simulink library "Fixed_Wing"  (R2023b)
settings: Solver=VariableStepAuto  StartTime=0.0  StopTime=10.0  RelTol=1e-3
values from neighbouring files (symbols this model uses):
  X8_lat_da_p_tf = X8_lat_p_tf(1)    [main.m]
  X8_lat_da_r_tf = X8_lat_r_tf(1)    [main.m]
  X8_lon_de_q_tf = X8_lon_q_tf(1)    [main.m]
  X8_lon_th_u_tf = X8_lon_u_tf(2)    [main.m]
  X8_lon_th_w_tf = X8_lon_w_tf(2)    [main.m]
undefined symbols (not defined in the file or in its folder): alpha, beta, env, init, k_phi, k_theta, k_Va, X8
libraries: $bdroot x16, simulink x2
(part 1 of 2)
settings Model: Creator=TigerWuu  LastModifiedBy=NCS

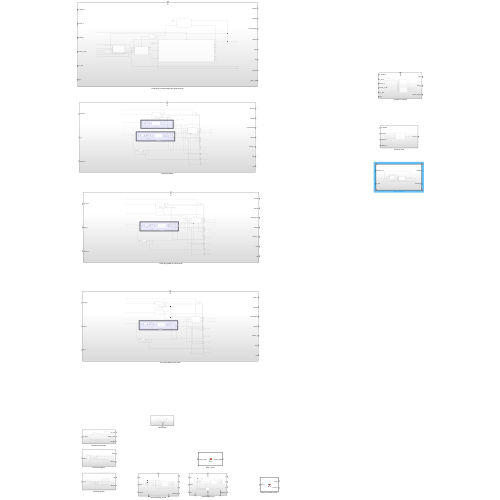
[thumbnail: Simulink's stored preview of the top-level diagram]
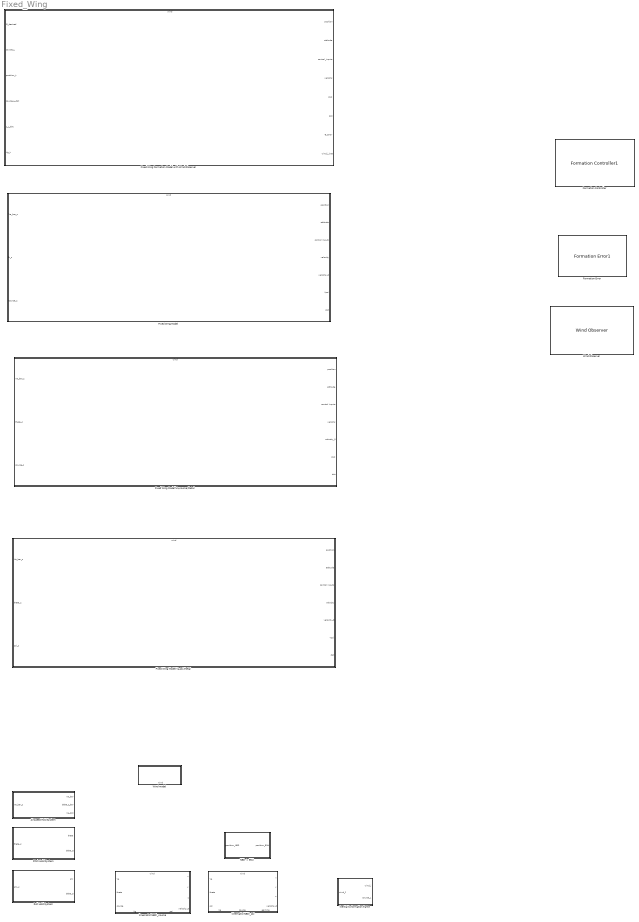
== system Fixed_Wing ==
  Airspeed Hold System : Subsystem
  Fixed Wing Formation Model with Wind Observer : Subsystem
      settings: PortSchema="{\"entries\":[{\"content\":{\"sides\":[{\"content\":{\"connectorIds\":[\"In1\",\"In2\",\"In3\",\"In4\",\"In5\",\"In6\"]},\"type\":\"ConnectorPlacement.EquallySpacedRectSide\",\"uuid\":\"527b8280-b7bb-4bbf-b75e-797629a1d02f\"},{\"content\":{\"connectorIds\":[\"Out1\",\"Out2\",\"Out3\",\"Out4\",\"Out5\",\"Out6\",\"Out7\",\"Out8\"],\"side\":\"RIGHT\"},\"type\":\"ConnectorPlacement.EquallySpacedRectSide\",\"uuid\":\"83651618-4cce-4797-8c5d-5752aadadd0e\"},{\"content\":{\"connectorIds\":[\"In7\"],\"side\":\"TOP\"},\"type\":\"ConnectorPlacement.EquallySpacedRectSide\",\"uuid\":\"91f129b3-c1c6-46ff-9e73-d368da7d167a\"}]},\"type\":\"ConnectorPlacement.EquallySpacedConnector\",\"uuid\":\"d5eae0c8-1f9e-4313-b74c-0f7e22e43491\"}],\"packageUris\":[\"http://schema.mathworks.com/mf0/Connector/R2020b\"],\"version\":\"1.0\"}"
  Fixed Wing Model : Subsystem
      settings: PortSchema="{\"entries\":[{\"content\":{\"sides\":[{\"content\":{\"connectorIds\":[\"In1\",\"In2\",\"In3\"]},\"type\":\"ConnectorPlacement.EquallySpacedRectSide\",\"uuid\":\"491080cc-ba33-4dca-9b37-922a1b131a7c\"},{\"content\":{\"connectorIds\":[\"Out1\",\"Out2\",\"Out3\",\"Out4\",\"Out5\",\"Out6\",\"Out7\"],\"side\":\"RIGHT\"},\"type\":\"ConnectorPlacement.EquallySpacedRectSide\",\"uuid\":\"e4e8ca81-264a-41b3-9d62-a2cb565f7b79\"},{\"content\":{\"connectorIds\":[\"In4\"],\"side\":\"TOP\"},\"type\":\"ConnectorPlacement.EquallySpacedRectSide\",\"uuid\":\"52444ebc-de17-4d3c-95e2-2270054ae63e\"},{\"content\":{\"side\":\"BOTTOM\"},\"type\":\"ConnectorPlacement.EquallySpacedRectSide\",\"uuid\":\"cd38afea-0687-422f-bcb3-a9854084c98f\"}]},\"type\":\"ConnectorPlacement.EquallySpacedConnector\",\"uuid\":\"020d1068-73e8-421c-b651-66bcdf43a07b\"}],\"packageUris\":[\"http://schema.mathworks.com/mf0/Connector/R2020b\"],\"version\":\"1.0\"}"
  Fixed Wing Model(Va,course,theta) : Subsystem
      settings: PortSchema="{\"entries\":[{\"content\":{\"sides\":[{\"content\":{\"connectorIds\":[\"In1\",\"In2\",\"In3\"]},\"type\":\"ConnectorPlacement.EquallySpacedRectSide\",\"uuid\":\"491080cc-ba33-4dca-9b37-922a1b131a7c\"},{\"content\":{\"connectorIds\":[\"Out1\",\"Out2\",\"Out3\",\"Out4\",\"Out5\",\"Out6\",\"Out7\"],\"side\":\"RIGHT\"},\"type\":\"ConnectorPlacement.EquallySpacedRectSide\",\"uuid\":\"e4e8ca81-264a-41b3-9d62-a2cb565f7b79\"},{\"content\":{\"connectorIds\":[\"In4\"],\"side\":\"TOP\"},\"type\":\"ConnectorPlacement.EquallySpacedRectSide\",\"uuid\":\"52444ebc-de17-4d3c-95e2-2270054ae63e\"},{\"content\":{\"side\":\"BOTTOM\"},\"type\":\"ConnectorPlacement.EquallySpacedRectSide\",\"uuid\":\"cd38afea-0687-422f-bcb3-a9854084c98f\"}]},\"type\":\"ConnectorPlacement.EquallySpacedConnector\",\"uuid\":\"020d1068-73e8-421c-b651-66bcdf43a07b\"}],\"packageUris\":[\"http://schema.mathworks.com/mf0/Connector/R2020b\"],\"version\":\"1.0\"}"
  Fixed Wing Model(Va,psi,theta) : Subsystem
      settings: PortSchema="{\"entries\":[{\"content\":{\"sides\":[{\"content\":{\"connectorIds\":[\"In1\",\"In2\",\"In3\"]},\"type\":\"ConnectorPlacement.EquallySpacedRectSide\",\"uuid\":\"491080cc-ba33-4dca-9b37-922a1b131a7c\"},{\"content\":{\"connectorIds\":[\"Out1\",\"Out2\",\"Out3\",\"Out4\",\"Out5\",\"Out6\",\"Out7\"],\"side\":\"RIGHT\"},\"type\":\"ConnectorPlacement.EquallySpacedRectSide\",\"uuid\":\"e4e8ca81-264a-41b3-9d62-a2cb565f7b79\"},{\"content\":{\"connectorIds\":[\"In4\"],\"side\":\"TOP\"},\"type\":\"ConnectorPlacement.EquallySpacedRectSide\",\"uuid\":\"52444ebc-de17-4d3c-95e2-2270054ae63e\"},{\"content\":{\"side\":\"BOTTOM\"},\"type\":\"ConnectorPlacement.EquallySpacedRectSide\",\"uuid\":\"cd38afea-0687-422f-bcb3-a9854084c98f\"}]},\"type\":\"ConnectorPlacement.EquallySpacedConnector\",\"uuid\":\"020d1068-73e8-421c-b651-66bcdf43a07b\"}],\"packageUris\":[\"http://schema.mathworks.com/mf0/Connector/R2020b\"],\"version\":\"1.0\"}"
  Formation Controller : $bdroot/Fixed Wing Formation Model with Wind Observer/Formation Controller1  SystemSampleTime=-1  VariantActivationTime=update diagram  AllowFlexibleInterface=on  Latency=0  AutoFrameSizeCalculation=off
      settings: PortSchema="{\"entries\":[{\"content\":{\"sides\":[{\"content\":{\"connectorIds\":[\"In1\",\"In2\",\"In3\",\"In4\",\"In5\",\"In6\"]},\"type\":\"ConnectorPlacement.EquallySpacedRectSide\",\"uuid\":\"9c389f85-23f7-4ad0-9870-58a1e0934639\"},{\"content\":{\"connectorIds\":[\"Out1\",\"Out2\",\"Out3\"],\"side\":\"RIGHT\"},\"type\":\"ConnectorPlacement.EquallySpacedRectSide\",\"uuid\":\"ce3247c4-1bae-44d3-b9da-13662f8788fa\"},{\"content\":{\"connectorIds\":[\"In7\"],\"side\":\"TOP\"},\"type\":\"ConnectorPlacement.EquallySpacedRectSide\",\"uuid\":\"1a627aed-9846-48b6-b280-b2fda66f57fb\"}]},\"type\":\"ConnectorPlacement.EquallySpacedConnector\",\"uuid\":\"4ccca4c3-7c97-47a5-8a1e-b96349422d36\"}],\"packageUris\":[\"http://schema.mathworks.com/mf0/Connector/R2020b\"],\"version\":\"1.0\"}"
  Formation Error : $bdroot/Fixed Wing Formation Model with Wind Observer/Formation Error1  SystemSampleTime=-1  VariantActivationTime=update diagram  AllowFlexibleInterface=on  Latency=0  AutoFrameSizeCalculation=off
  Inertial to formation frame : MATLAB Function  TreatAsAtomicUnit=on
  "NED -> ENU" : MATLAB Function  TreatAsAtomicUnit=on
  "Pitch Hold System " : Subsystem
      settings: ModelCloseFcn=function
  Roll Hold System : Subsystem
      settings: ModelCloseFcn=function
  Wind Observer : $bdroot/Fixed Wing Formation Model with Wind Observer/Wind Observer  SystemSampleTime=-1  VariantActivationTime=update diagram  AllowFlexibleInterface=on  Latency=0  AutoFrameSizeCalculation=off
  Wind model : Subsystem
      settings: PortSchema="{\"entries\":[{\"content\":{\"sides\":[{\"content\":{},\"type\":\"ConnectorPlacement.EquallySpacedRectSide\",\"uuid\":\"19ef0eb7-c626-45ec-b76b-8668fc024824\"},{\"content\":{\"side\":\"RIGHT\"},\"type\":\"ConnectorPlacement.EquallySpacedRectSide\",\"uuid\":\"89e72569-ab94-4162-a6e2-b425ef08f724\"},{\"content\":{\"side\":\"TOP\"},\"type\":\"ConnectorPlacement.EquallySpacedRectSide\",\"uuid\":\"6d9409e9-6822-4cd9-902f-e5665cb68433\"},{\"content\":{\"connectorIds\":[\"Out1\"],\"side\":\"BOTTOM\"},\"type\":\"ConnectorPlacement.EquallySpacedRectSide\",\"uuid\":\"39a83352-0924-44fa-be5d-94a7c28bbbf3\"}]},\"type\":\"ConnectorPlacement.EquallySpacedConnector\",\"uuid\":\"6cf6ae00-ef23-42a2-99b2-ca60e191fb03\"}],\"packageUris\":[\"http://schema.mathworks.com/mf0/Connector/R2020b\"],\"version\":\"1.0\"}"
  kinematic(NED)_course : Subsystem
      settings: PortSchema="{\"entries\":[{\"content\":{\"sides\":[{\"content\":{\"connectorIds\":[\"In1\",\"In2\",\"In3\"]},\"type\":\"ConnectorPlacement.EquallySpacedRectSide\",\"uuid\":\"96d967d8-b822-4ab1-b08a-27adc20d5833\"},{\"content\":{\"connectorIds\":[\"Out1\",\"Out2\",\"Out3\",\"Out4\"],\"side\":\"RIGHT\"},\"type\":\"ConnectorPlacement.EquallySpacedRectSide\",\"uuid\":\"505a36c9-cae2-422c-97bf-34d37872a31d\"},{\"content\":{\"connectorIds\":[\"In4\"],\"side\":\"TOP\"},\"type\":\"ConnectorPlacement.EquallySpacedRectSide\",\"uuid\":\"7bc53155-5df6-4b6a-9756-725497693b0a\"},{\"content\":{\"connectorIds\":[\"Out5\",\"Out6\"],\"side\":\"BOTTOM\"},\"type\":\"ConnectorPlacement.EquallySpacedRectSide\",\"uuid\":\"7777b465-a27e-4b61-9b89-f3b8fa4654d1\"}]},\"type\":\"ConnectorPlacement.EquallySpacedConnector\",\"uuid\":\"2150a812-5a4a-4a29-9c93-d226d95b2326\"}],\"packageUris\":[\"http://schema.mathworks.com/mf0/Connector/R2020b\"],\"version\":\"1.0\"}"
  kinematic(NED)_psi : Subsystem
      settings: PortSchema="{\"entries\":[{\"content\":{\"sides\":[{\"content\":{\"connectorIds\":[\"In1\",\"In2\",\"In3\"]},\"type\":\"ConnectorPlacement.EquallySpacedRectSide\",\"uuid\":\"96d967d8-b822-4ab1-b08a-27adc20d5833\"},{\"content\":{\"connectorIds\":[\"Out1\",\"Out2\",\"Out3\",\"Out4\"],\"side\":\"RIGHT\"},\"type\":\"ConnectorPlacement.EquallySpacedRectSide\",\"uuid\":\"505a36c9-cae2-422c-97bf-34d37872a31d\"},{\"content\":{\"connectorIds\":[\"In4\"],\"side\":\"TOP\"},\"type\":\"ConnectorPlacement.EquallySpacedRectSide\",\"uuid\":\"7bc53155-5df6-4b6a-9756-725497693b0a\"},{\"content\":{\"connectorIds\":[\"Out5\",\"Out6\",\"Out7\"],\"side\":\"BOTTOM\"},\"type\":\"ConnectorPlacement.EquallySpacedRectSide\",\"uuid\":\"7777b465-a27e-4b61-9b89-f3b8fa4654d1\"}]},\"type\":\"ConnectorPlacement.EquallySpacedConnector\",\"uuid\":\"2150a812-5a4a-4a29-9c93-d226d95b2326\"}],\"packageUris\":[\"http://schema.mathworks.com/mf0/Connector/R2020b\"],\"version\":\"1.0\"}"

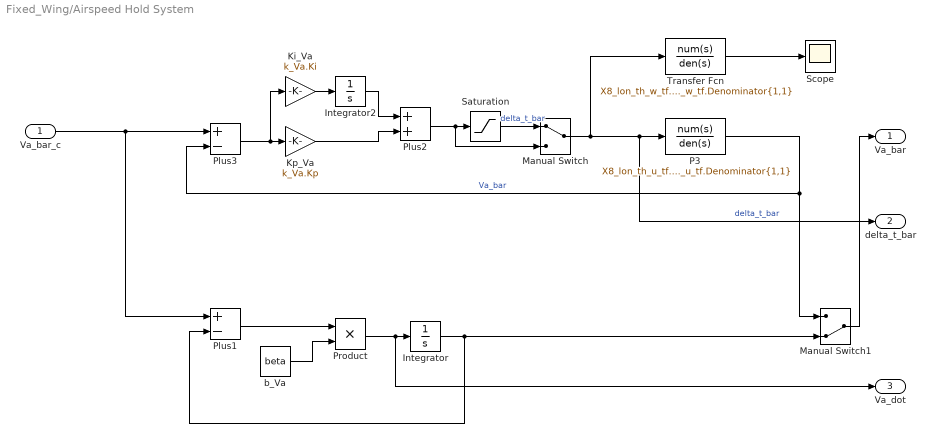
== system Fixed_Wing/Airspeed Hold System ==
  Va_bar_c : Inport
  Integrator : Integrator
  Integrator2 : Integrator
  Ki_Va : Gain  Gain=k_Va.Ki
  Kp_Va : Gain  Gain=k_Va.Kp
  Manual Switch : ManualSwitch
  Manual Switch1 : ManualSwitch  CurrentSetting=0
  P3 : TransferFcn  Numerator=X8_lon_th_u_tf.Numerator{1,1}  Denominator=X8_lon_th_u_tf.Denominator{1,1}
  Plus1 : Sum  Inputs=+-
  Plus2 : Sum
  Plus3 : Sum  Inputs=+-
  Product : Product
  Saturation : Saturate  UpperLimit=X8.delta.t_max-X8.delta.t_star  LowerLimit=X8.delta.t_min -X8.delta.t_star  LinearizeAsGain=off
  Scope : Scope
  Transfer Fcn : TransferFcn  Numerator=X8_lon_th_w_tf.Numerator{1,1}  Denominator=X8_lon_th_w_tf.Denominator{1,1}
  b_Va : Constant  Value=beta
  Va_bar : Outport
  delta_t_bar : Outport  Port=2
  Va_dot : Outport  Port=3
  wires:
  Ki_Va/1 -> Integrator2/1
  Plus3/1 -> Ki_Va/1, Kp_Va/1
  Kp_Va/1 -> Plus2/2
  Plus2/1 -> Manual Switch/2, Saturation/1
  Integrator2/1 -> Plus2/1
  P3/1 -> Manual Switch1/1, Plus3/2  "Va_bar"
  Manual Switch/1 -> Transfer Fcn/1, P3/1, delta_t_bar/1  "delta_t_bar"
  Transfer Fcn/1 -> Scope/1
  Saturation/1 -> Manual Switch/1  "delta_t_bar"
  Plus1/1 -> Product/1
  b_Va/1 -> Product/2
  Product/1 -> Va_dot/1, Integrator/1
  Integrator/1 -> Manual Switch1/2, Plus1/2
  Va_bar_c/1 -> Plus1/1, Plus3/1
  Manual Switch1/1 -> Va_bar/1

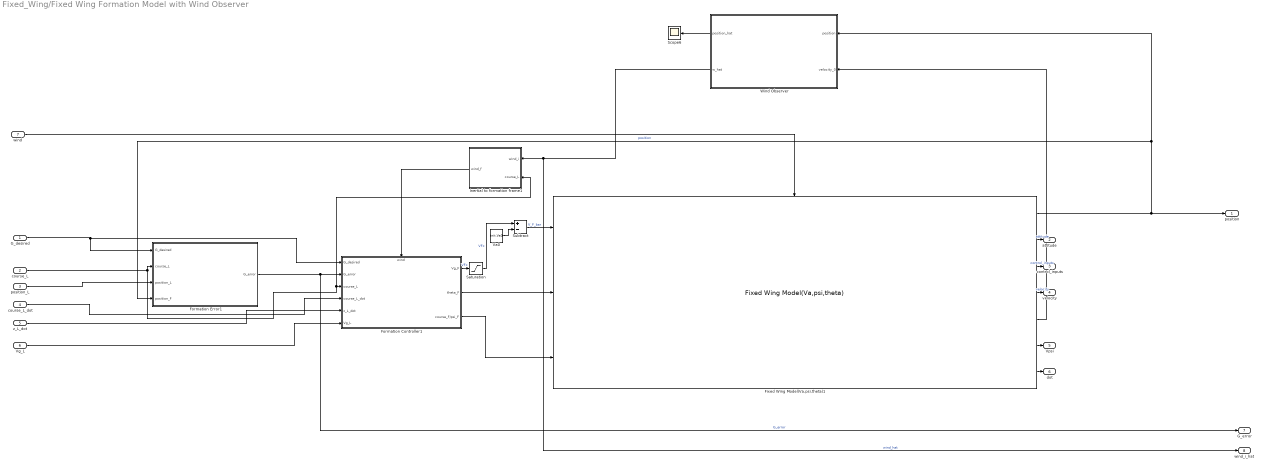
== system Fixed_Wing/Fixed Wing Formation Model with Wind Observer ==
  G_desired : Inport
  course_L : Inport  Port=2
  position_L : Inport  Port=3
  course_L_dot : Inport  Port=4
  z_L_dot : Inport  Port=5
  Vg_L : Inport  Port=6
  wind : Inport  Port=7
  Fixed Wing Model(Va,psi,theta)1 : $bdroot/Fixed Wing Model(Va,psi,theta)  SystemSampleTime=-1  VariantActivationTime=update diagram  AllowFlexibleInterface=on  Latency=0  AutoFrameSizeCalculation=off
      link override Ki_course: Gain=0
      settings: PortSchema="{\"entries\":[{\"content\":{\"sides\":[{\"content\":{\"connectorIds\":[\"In1\",\"In2\",\"In3\"]},\"type\":\"ConnectorPlacement.EquallySpacedRectSide\",\"uuid\":\"491080cc-ba33-4dca-9b37-922a1b131a7c\"},{\"content\":{\"connectorIds\":[\"Out1\",\"Out2\",\"Out3\",\"Out4\",\"Out5\",\"Out6\",\"Out7\"],\"side\":\"RIGHT\"},\"type\":\"ConnectorPlacement.EquallySpacedRectSide\",\"uuid\":\"e4e8ca81-264a-41b3-9d62-a2cb565f7b79\"},{\"content\":{\"connectorIds\":[\"In4\"],\"side\":\"TOP\"},\"type\":\"ConnectorPlacement.EquallySpacedRectSide\",\"uuid\":\"52444ebc-de17-4d3c-95e2-2270054ae63e\"},{\"content\":{\"side\":\"BOTTOM\"},\"type\":\"ConnectorPlacement.EquallySpacedRectSide\",\"uuid\":\"cd38afea-0687-422f-bcb3-a9854084c98f\"}]},\"type\":\"ConnectorPlacement.EquallySpacedConnector\",\"uuid\":\"020d1068-73e8-421c-b651-66bcdf43a07b\"}],\"packageUris\":[\"http://schema.mathworks.com/mf0/Connector/R2020b\"],\"version\":\"1.0\"}"
  Formation Controller1 : Subsystem
      settings: PortSchema="{\"entries\":[{\"content\":{\"sides\":[{\"content\":{\"connectorIds\":[\"In1\",\"In2\",\"In3\",\"In4\",\"In5\",\"In6\"]},\"type\":\"ConnectorPlacement.EquallySpacedRectSide\",\"uuid\":\"9c389f85-23f7-4ad0-9870-58a1e0934639\"},{\"content\":{\"connectorIds\":[\"Out1\",\"Out2\",\"Out3\"],\"side\":\"RIGHT\"},\"type\":\"ConnectorPlacement.EquallySpacedRectSide\",\"uuid\":\"ce3247c4-1bae-44d3-b9da-13662f8788fa\"},{\"content\":{\"connectorIds\":[\"In7\"],\"side\":\"TOP\"},\"type\":\"ConnectorPlacement.EquallySpacedRectSide\",\"uuid\":\"1a627aed-9846-48b6-b280-b2fda66f57fb\"}]},\"type\":\"ConnectorPlacement.EquallySpacedConnector\",\"uuid\":\"4ccca4c3-7c97-47a5-8a1e-b96349422d36\"}],\"packageUris\":[\"http://schema.mathworks.com/mf0/Connector/R2020b\"],\"version\":\"1.0\"}"
  Formation Error1 : Subsystem
  Inertial to formation frame1 : MATLAB Function  TreatAsAtomicUnit=on
  Saturation : Saturate  UpperLimit=28  LowerLimit=12
  Scope6 : Scope
  Subtract : Sum  Inputs=+-
  Va0 : Constant  Value=init.Va0
  Wind Observer : Subsystem
  position : Outport
  attitude : Outport  Port=2
  control_inputs : Outport  Port=3
  velocity : Outport  Port=4
  Vpsi : Outport  Port=5
  dot : Outport  Port=6
  G_error : Outport  Port=7
  wind_i_hat : Outport  Port=8
  wires:
  Wind Observer/1(position_hat) -> Scope6/1
  Va0/1 -> Subtract/2
  Fixed Wing Model(Va,psi,theta)1/2 -> attitude/1  "attitude"
  Fixed Wing Model(Va,psi,theta)1/1 -> position/1, Formation Error1/4(position_F), Wind Observer/1(position)  "position"
  wind/1 -> Fixed Wing Model(Va,psi,theta)1/4
  position_L/1 -> Formation Error1/3(position_L)
  Vg_L/1 -> Formation Controller1/6(Vg_L)
  Fixed Wing Model(Va,psi,theta)1/7 -> dot/1
  Formation Controller1/2(theta_F) -> Fixed Wing Model(Va,psi,theta)1/2
  Formation Error1/1(G_error) -> G_error/1, Formation Controller1/2(G_error)  "G_error"
  Formation Controller1/1(Vg_F) -> Saturation/1  "VFc"
  Subtract/1 -> Fixed Wing Model(Va,psi,theta)1/1  "V_F_bar"
  Formation Controller1/3(course_F/psi_F) -> Fixed Wing Model(Va,psi,theta)1/3
  Fixed Wing Model(Va,psi,theta)1/3 -> control_inputs/1  "control_inputs"
  Wind Observer/2(w_hat) -> wind_i_hat/1, Inertial to formation frame1/1(wind_i)  "wind_hat"
  course_L/1 -> Inertial to formation frame1/2(course_L), Formation Controller1/3(course_L), Formation Error1/2(course_L)
  Fixed Wing Model(Va,psi,theta)1/4 -> velocity/1  "velocity"
  Inertial to formation frame1/1(wind_f) -> Formation Controller1/7(wind)
  Saturation/1 -> Subtract/1  "VFc"
  Fixed Wing Model(Va,psi,theta)1/5 -> Wind Observer/2(velocity_0)
  z_L_dot/1 -> Formation Controller1/5(z_L_dot)
  course_L_dot/1 -> Formation Controller1/4(course_L_dot)
  G_desired/1 -> Formation Error1/1(G_desired), Formation Controller1/1(G_desired)
  Fixed Wing Model(Va,psi,theta)1/6 -> Vpsi/1

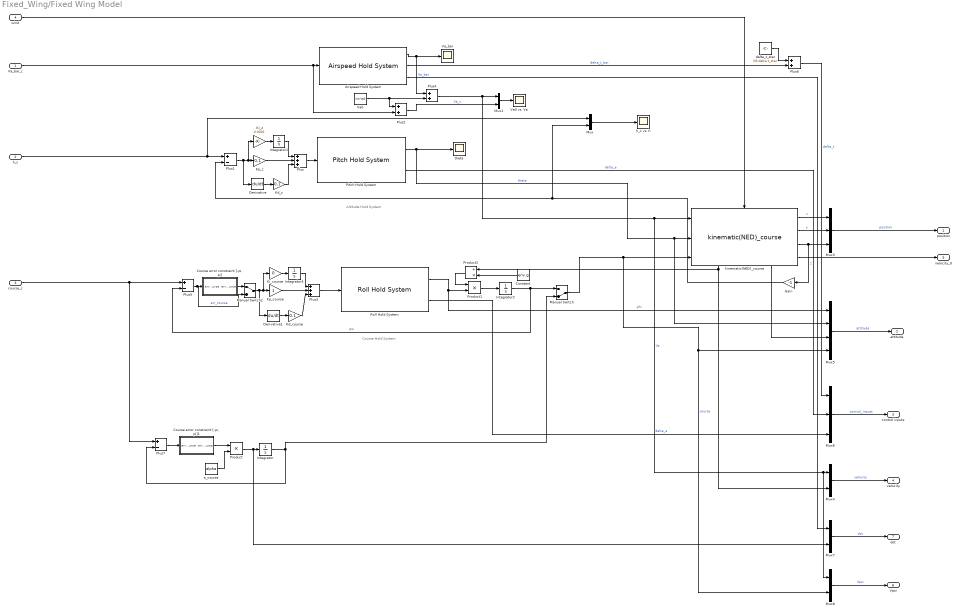
== system Fixed_Wing/Fixed Wing Model ==
  note: Course Hold System
  note: Altitude Hold System
  Va_bar_c : Inport
  h_c : Inport  Port=2
  course_c : Inport  Port=3
  wind : Inport  Port=4
  Airspeed Hold System : $bdroot/Airspeed Hold System  SystemSampleTime=-1  VariantActivationTime=update diagram  AllowFlexibleInterface=on  Latency=0  AutoFrameSizeCalculation=off
      link override b_Va: Value=beta
  Constant : Constant  Value=env.g
  "Course error constraint [-pi, pi]" : MATLAB Function  TreatAsAtomicUnit=on
  "Course error constraint [-pi, pi]1" : MATLAB Function  TreatAsAtomicUnit=on
  Derivative : Derivative
  Derivative1 : Derivative
  Gain : Gain  Gain=-1
  Integrator : Integrator
  Integrator1 : Integrator
  Integrator2 : Integrator  InitialCondition=init.course0
  Integrator3 : Integrator
  Kd_course : Gain  Gain=0.1
  Kd_z : Gain  Gain=0.1
  Ki_course : Gain  Gain=0
  Ki_z : Gain  Gain=0.0001
  Kp_course : Gain
  Kp_z : Gain  Gain=0.1
  Manual Switch : ManualSwitch  CurrentSetting=0
  Manual Switch2 : ManualSwitch
  Mux{,1,4,7..8} (5 alike) : Mux  Inputs=2
  Mux3 : Mux  Inputs=3
  Mux5 : Mux
  Mux6 : Mux  Inputs=3
  "Pitch Hold System " : $bdroot/Pitch Hold System   SystemSampleTime=-1  VariantActivationTime=update diagram  AllowFlexibleInterface=on  Latency=0  AutoFrameSizeCalculation=off
  Plus : Sum  Inputs=+++
  Plus1 : Sum  Inputs=+-
  Plus2 : Sum
  Plus3 : Sum  Inputs=+++
  Plus4 : Sum
  Plus5 : Sum  Inputs=+-
  Plus6 : Sum
  Plus7 : Sum  Inputs=+-
  Product : Product
  Product1 : Product
  Product2 : Product  Inputs=/*
  Roll Hold System : $bdroot/Roll Hold System  SystemSampleTime=-1  VariantActivationTime=update diagram  AllowFlexibleInterface=on  Latency=0  AutoFrameSizeCalculation=off
  Va0 : Constant  Value=init.Va0
  Va0 vs. Va : Scope
  Va_bar : Scope
  a_course : Constant  Value=alpha
  delta_t_star : Constant  Value=X8.delta.t_star
  h_c vs. h : Scope
  kinematic(NED)_course : $bdroot/kinematic(NED)_course  SystemSampleTime=-1  VariantActivationTime=update diagram  AllowFlexibleInterface=on  Latency=0  AutoFrameSizeCalculation=off
      settings: PortSchema="{\"entries\":[{\"content\":{\"sides\":[{\"content\":{\"connectorIds\":[\"In1\",\"In2\",\"In3\"]},\"type\":\"ConnectorPlacement.EquallySpacedRectSide\",\"uuid\":\"96d967d8-b822-4ab1-b08a-27adc20d5833\"},{\"content\":{\"connectorIds\":[\"Out1\",\"Out2\",\"Out3\",\"Out4\"],\"side\":\"RIGHT\"},\"type\":\"ConnectorPlacement.EquallySpacedRectSide\",\"uuid\":\"505a36c9-cae2-422c-97bf-34d37872a31d\"},{\"content\":{\"connectorIds\":[\"In4\"],\"side\":\"TOP\"},\"type\":\"ConnectorPlacement.EquallySpacedRectSide\",\"uuid\":\"7bc53155-5df6-4b6a-9756-725497693b0a\"},{\"content\":{\"connectorIds\":[\"Out5\",\"Out6\"],\"side\":\"BOTTOM\"},\"type\":\"ConnectorPlacement.EquallySpacedRectSide\",\"uuid\":\"7777b465-a27e-4b61-9b89-f3b8fa4654d1\"}]},\"type\":\"ConnectorPlacement.EquallySpacedConnector\",\"uuid\":\"2150a812-5a4a-4a29-9c93-d226d95b2326\"}],\"packageUris\":[\"http://schema.mathworks.com/mf0/Connector/R2020b\"],\"version\":\"1.0\"}"
  theta : Scope
  position : Outport
  attitude : Outport  Port=2
  control inputs : Outport  Port=3
  velocity : Outport  Port=4
  velocity_0 : Outport  Port=5
  Vpsi : Outport  Port=6
  dot : Outport  Port=7
  wires:
  Integrator3/1 -> Plus3/1
  Integrator1/1 -> Plus/1
  kinematic(NED)_course/3 -> Gain/1, Mux3/3  "z"
  kinematic(NED)_course/1 -> Mux3/1  "x"
  Derivative1/1 -> Kd_course/1
  Constant/1 -> Product2/2
  Va0/1 -> Plus2/1, Plus4/2
  "Pitch Hold System "/1 -> kinematic(NED)_course/2, Mux5/2, theta/1  "theta"
  Kd_z/1 -> Plus/3
  kinematic(NED)_course/2 -> Mux3/2  "y"
  h_c/1 -> Mux/1, Plus1/1
  Plus1/1 -> Derivative/1, Ki_z/1, Kp_z/1
  Va_bar_c/1 -> Plus2/2, Airspeed Hold System/1
  Gain/1 -> Mux/2, Plus1/2
  Roll Hold System/2 -> Mux6/3  "delta_a"
  Kp_z/1 -> Plus/2
  Plus/1 -> "Pitch Hold System "/1
  Airspeed Hold System/2 -> Plus6/2  "delta_t_bar"
  Derivative/1 -> Kd_z/1
  "Pitch Hold System "/2 -> Mux6/2  "delta_e"
  Plus6/1 -> Mux6/1  "delta_t"
  Airspeed Hold System/1 -> Plus4/1, Va_bar/1  "Va_bar"
  delta_t_star/1 -> Plus6/1
  Mux3/1 -> position/1  "position"
  Ki_z/1 -> Integrator1/1
  Integrator2/1 -> Manual Switch/1, Plus5/2  "psi"
  Ki_course/1 -> Integrator3/1
  Product1/1 -> Integrator2/1
  Kp_course/1 -> Plus3/2
  Product2/1 -> Product1/1
  Plus5/1 -> Manual Switch2/2, "Course error constraint [-pi, pi]"/1("err_course ")  "err_course"
  Plus3/1 -> Roll Hold System/1
  Mux/1 -> h_c vs. h/1
  Plus4/1 -> Mux1/1, kinematic(NED)_course/1, Mux8/1, Mux4/1  "Va"
  Mux1/1 -> Va0 vs. Va/1
  kinematic(NED)_course/5 -> Mux4/2, Product2/1
  Mux6/1 -> control inputs/1  "control_inputs"
  Plus2/1 -> Mux1/2  "Va_c"
  Mux5/1 -> attitude/1  "attitude"
  Kd_course/1 -> Plus3/3
  Roll Hold System/1 -> Mux5/1, Product1/2  "phi"
  wind/1 -> kinematic(NED)_course/4
  Manual Switch2/1 -> Derivative1/1, Ki_course/1, Kp_course/1
  Mux4/1 -> velocity/1  "velocity"
  "Course error constraint [-pi, pi]"/1(err_course) -> Manual Switch2/1
  a_course/1 -> Product/2
  Product/1 -> Mux7/2, Integrator/1
  Integrator/1 -> Manual Switch/2, Plus7/2
  Plus7/1 -> "Course error constraint [-pi, pi]1"/1("err_course ")
  course_c/1 -> Plus5/1, Plus7/1
  "Course error constraint [-pi, pi]1"/1(err_course) -> Product/1
  Mux7/1 -> dot/1  "dot"
  Airspeed Hold System/3 -> Mux7/1
  Mux8/1 -> Vpsi/1  "Vpsi"
  Manual Switch/1 -> kinematic(NED)_course/3, Mux8/2, Mux5/4  "course"
  kinematic(NED)_course/4 -> velocity_0/1
  kinematic(NED)_course/6 -> Mux5/3

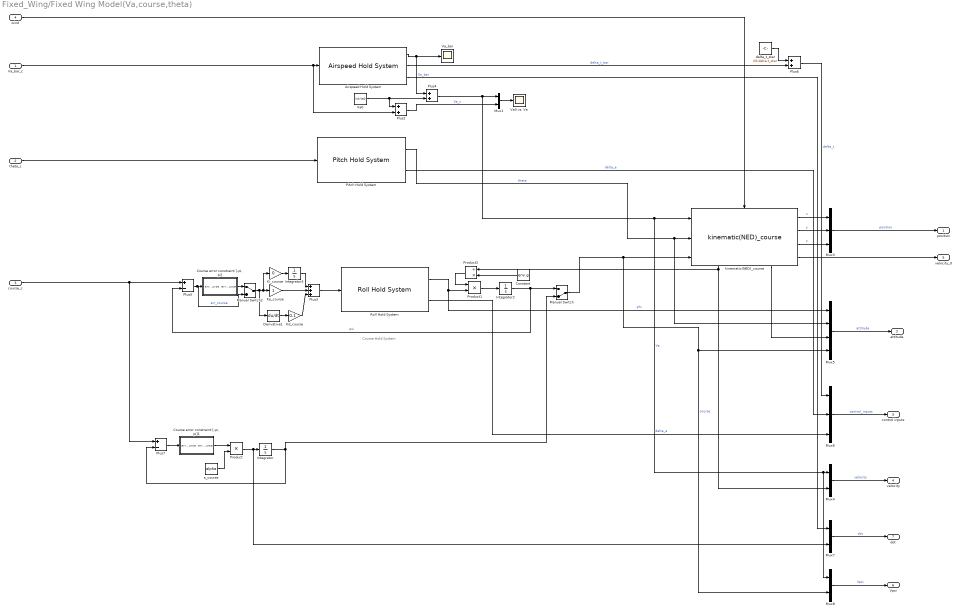
== system Fixed_Wing/Fixed Wing Model(Va,course,theta) ==
  note: Course Hold System
  Va_bar_c : Inport
  theta_c : Inport  Port=2
  course_c : Inport  Port=3
  wind : Inport  Port=4
  Airspeed Hold System : $bdroot/Airspeed Hold System  SystemSampleTime=-1  VariantActivationTime=update diagram  AllowFlexibleInterface=on  Latency=0  AutoFrameSizeCalculation=off
  Constant : Constant  Value=env.g
  "Course error constraint [-pi, pi]" : MATLAB Function  TreatAsAtomicUnit=on
  "Course error constraint [-pi, pi]1" : MATLAB Function  TreatAsAtomicUnit=on
  Derivative1 : Derivative
  Integrator : Integrator
  Integrator2 : Integrator  InitialCondition=init.course0
  Integrator3 : Integrator
  Kd_course : Gain  Gain=0.1
  Ki_course : Gain  Gain=0
  Kp_course : Gain
  Manual Switch : ManualSwitch  CurrentSetting=0
  Manual Switch2 : ManualSwitch
  Mux{1,4,7..8} (4 alike) : Mux  Inputs=2
  Mux3 : Mux  Inputs=3
  Mux5 : Mux
  Mux6 : Mux  Inputs=3
  "Pitch Hold System " : $bdroot/Pitch Hold System   SystemSampleTime=-1  VariantActivationTime=update diagram  AllowFlexibleInterface=on  Latency=0  AutoFrameSizeCalculation=off
  Plus2 : Sum
  Plus3 : Sum  Inputs=+++
  Plus4 : Sum
  Plus5 : Sum  Inputs=+-
  Plus6 : Sum
  Plus7 : Sum  Inputs=+-
  Product : Product
  Product1 : Product
  Product2 : Product  Inputs=/*
  Roll Hold System : $bdroot/Roll Hold System  SystemSampleTime=-1  VariantActivationTime=update diagram  AllowFlexibleInterface=on  Latency=0  AutoFrameSizeCalculation=off
  Va0 : Constant  Value=init.Va0
  Va0 vs. Va : Scope
  Va_bar : Scope
  a_course : Constant  Value=alpha
  delta_t_star : Constant  Value=X8.delta.t_star
  kinematic(NED)_course : $bdroot/kinematic(NED)_course  SystemSampleTime=-1  VariantActivationTime=update diagram  AllowFlexibleInterface=on  Latency=0  AutoFrameSizeCalculation=off
      settings: PortSchema="{\"entries\":[{\"content\":{\"sides\":[{\"content\":{\"connectorIds\":[\"In1\",\"In2\",\"In3\"]},\"type\":\"ConnectorPlacement.EquallySpacedRectSide\",\"uuid\":\"96d967d8-b822-4ab1-b08a-27adc20d5833\"},{\"content\":{\"connectorIds\":[\"Out1\",\"Out2\",\"Out3\",\"Out4\"],\"side\":\"RIGHT\"},\"type\":\"ConnectorPlacement.EquallySpacedRectSide\",\"uuid\":\"505a36c9-cae2-422c-97bf-34d37872a31d\"},{\"content\":{\"connectorIds\":[\"In4\"],\"side\":\"TOP\"},\"type\":\"ConnectorPlacement.EquallySpacedRectSide\",\"uuid\":\"7bc53155-5df6-4b6a-9756-725497693b0a\"},{\"content\":{\"connectorIds\":[\"Out5\",\"Out6\"],\"side\":\"BOTTOM\"},\"type\":\"ConnectorPlacement.EquallySpacedRectSide\",\"uuid\":\"7777b465-a27e-4b61-9b89-f3b8fa4654d1\"}]},\"type\":\"ConnectorPlacement.EquallySpacedConnector\",\"uuid\":\"2150a812-5a4a-4a29-9c93-d226d95b2326\"}],\"packageUris\":[\"http://schema.mathworks.com/mf0/Connector/R2020b\"],\"version\":\"1.0\"}"
  position : Outport
  attitude : Outport  Port=2
  control inputs : Outport  Port=3
  velocity : Outport  Port=4
  velocity_0 : Outport  Port=5
  Vpsi : Outport  Port=6
  dot : Outport  Port=7
  wires:
  Integrator3/1 -> Plus3/1
  kinematic(NED)_course/3 -> Mux3/3  "z"
  kinematic(NED)_course/1 -> Mux3/1  "x"
  Derivative1/1 -> Kd_course/1
  Constant/1 -> Product2/2
  Va0/1 -> Plus2/1, Plus4/2
  "Pitch Hold System "/1 -> kinematic(NED)_course/2, Mux5/2  "theta"
  kinematic(NED)_course/2 -> Mux3/2  "y"
  Va_bar_c/1 -> Plus2/2, Airspeed Hold System/1
  Roll Hold System/2 -> Mux6/3  "delta_a"
  theta_c/1 -> "Pitch Hold System "/1
  Airspeed Hold System/2 -> Plus6/2  "delta_t_bar"
  "Pitch Hold System "/2 -> Mux6/2  "delta_e"
  Plus6/1 -> Mux6/1  "delta_t"
  Airspeed Hold System/1 -> Plus4/1, Va_bar/1  "Va_bar"
  delta_t_star/1 -> Plus6/1
  Mux3/1 -> position/1  "position"
  Integrator2/1 -> Manual Switch/1, Plus5/2  "psi"
  Ki_course/1 -> Integrator3/1
  Product1/1 -> Integrator2/1
  Kp_course/1 -> Plus3/2
  Product2/1 -> Product1/1
  Plus5/1 -> Manual Switch2/2, "Course error constraint [-pi, pi]"/1("err_course ")  "err_course"
  Plus3/1 -> Roll Hold System/1
  Plus4/1 -> Mux1/1, kinematic(NED)_course/1, Mux8/1, Mux4/1  "Va"
  Mux1/1 -> Va0 vs. Va/1
  kinematic(NED)_course/5 -> Mux4/2, Product2/1
  Mux6/1 -> control inputs/1  "control_inputs"
  Plus2/1 -> Mux1/2  "Va_c"
  Mux5/1 -> attitude/1  "attitude"
  Kd_course/1 -> Plus3/3
  Roll Hold System/1 -> Mux5/1, Product1/2  "phi"
  wind/1 -> kinematic(NED)_course/4
  Manual Switch2/1 -> Derivative1/1, Ki_course/1, Kp_course/1
  Mux4/1 -> velocity/1  "velocity"
  "Course error constraint [-pi, pi]"/1(err_course) -> Manual Switch2/1
  a_course/1 -> Product/2
  Product/1 -> Mux7/2, Integrator/1
  Integrator/1 -> Manual Switch/2, Plus7/2
  Plus7/1 -> "Course error constraint [-pi, pi]1"/1("err_course ")
  course_c/1 -> Plus5/1, Plus7/1
  "Course error constraint [-pi, pi]1"/1(err_course) -> Product/1
  Mux7/1 -> dot/1  "dot"
  Airspeed Hold System/3 -> Mux7/1
  Mux8/1 -> Vpsi/1  "Vpsi"
  Manual Switch/1 -> kinematic(NED)_course/3, Mux8/2, Mux5/4  "course"
  kinematic(NED)_course/4 -> velocity_0/1
  kinematic(NED)_course/6 -> Mux5/3

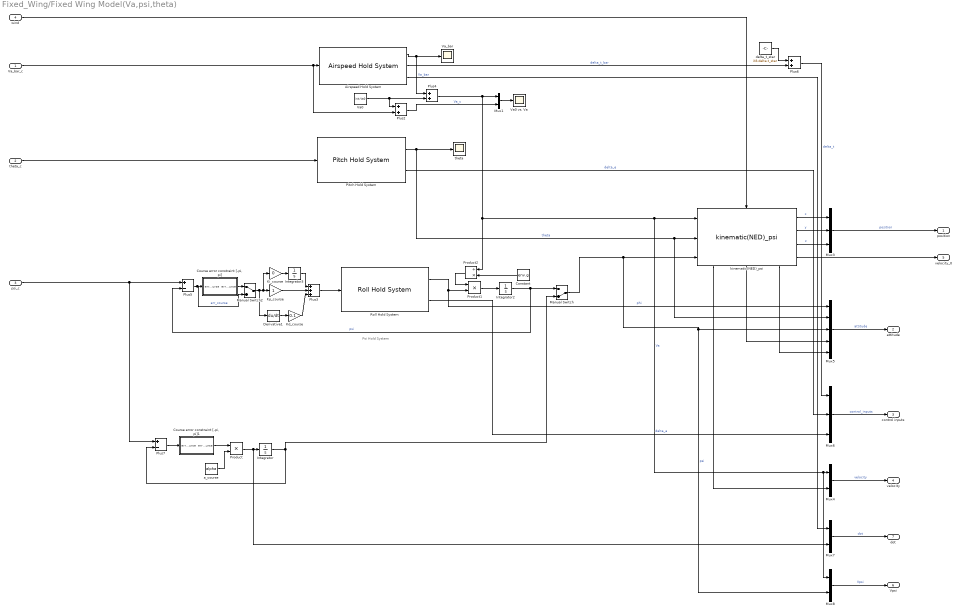
== system Fixed_Wing/Fixed Wing Model(Va,psi,theta) ==
  note: Psi Hold System
  Va_bar_c : Inport
  theta_c : Inport  Port=2
  psi_c : Inport  Port=3
  wind : Inport  Port=4
  Airspeed Hold System : $bdroot/Airspeed Hold System  SystemSampleTime=-1  VariantActivationTime=update diagram  AllowFlexibleInterface=on  Latency=0  AutoFrameSizeCalculation=off
  Constant : Constant  Value=env.g
  "Course error constraint [-pi, pi]" : MATLAB Function  TreatAsAtomicUnit=on
  "Course error constraint [-pi, pi]1" : MATLAB Function  TreatAsAtomicUnit=on
  Derivative1 : Derivative
  Integrator : Integrator
  Integrator2 : Integrator  InitialCondition=init.course0
  Integrator3 : Integrator
  Kd_course : Gain  Gain=0.1
  Ki_course : Gain  Gain=0
  Kp_course : Gain
  Manual Switch : ManualSwitch  CurrentSetting=0
  Manual Switch2 : ManualSwitch
  Mux{1,4,7..8} (4 alike) : Mux  Inputs=2
  Mux3 : Mux  Inputs=3
  Mux5 : Mux  Inputs=5
  Mux6 : Mux  Inputs=3
  "Pitch Hold System " : $bdroot/Pitch Hold System   SystemSampleTime=-1  VariantActivationTime=update diagram  AllowFlexibleInterface=on  Latency=0  AutoFrameSizeCalculation=off
  Plus2 : Sum
  Plus3 : Sum  Inputs=+++
  Plus4 : Sum
  Plus5 : Sum  Inputs=+-
  Plus6 : Sum
  Plus7 : Sum  Inputs=+-
  Product : Product
  Product1 : Product
  Product2 : Product  Inputs=/*
  Roll Hold System : $bdroot/Roll Hold System  SystemSampleTime=-1  VariantActivationTime=update diagram  AllowFlexibleInterface=on  Latency=0  AutoFrameSizeCalculation=off
  Va0 : Constant  Value=init.Va0
  Va0 vs. Va : Scope
  Va_bar : Scope
  a_course : Constant  Value=alpha
  delta_t_star : Constant  Value=X8.delta.t_star
  kinematic(NED)_psi : $bdroot/kinematic(NED)_psi  SystemSampleTime=-1  VariantActivationTime=update diagram  AllowFlexibleInterface=on  Latency=0  AutoFrameSizeCalculation=off
      settings: PortSchema="{\"entries\":[{\"content\":{\"sides\":[{\"content\":{\"connectorIds\":[\"In1\",\"In2\",\"In3\"]},\"type\":\"ConnectorPlacement.EquallySpacedRectSide\",\"uuid\":\"96d967d8-b822-4ab1-b08a-27adc20d5833\"},{\"content\":{\"connectorIds\":[\"Out1\",\"Out2\",\"Out3\",\"Out4\"],\"side\":\"RIGHT\"},\"type\":\"ConnectorPlacement.EquallySpacedRectSide\",\"uuid\":\"505a36c9-cae2-422c-97bf-34d37872a31d\"},{\"content\":{\"connectorIds\":[\"In4\"],\"side\":\"TOP\"},\"type\":\"ConnectorPlacement.EquallySpacedRectSide\",\"uuid\":\"7bc53155-5df6-4b6a-9756-725497693b0a\"},{\"content\":{\"connectorIds\":[\"Out5\",\"Out6\",\"Out7\"],\"side\":\"BOTTOM\"},\"type\":\"ConnectorPlacement.EquallySpacedRectSide\",\"uuid\":\"7777b465-a27e-4b61-9b89-f3b8fa4654d1\"}]},\"type\":\"ConnectorPlacement.EquallySpacedConnector\",\"uuid\":\"2150a812-5a4a-4a29-9c93-d226d95b2326\"}],\"packageUris\":[\"http://schema.mathworks.com/mf0/Connector/R2020b\"],\"version\":\"1.0\"}"
  theta : Scope
  position : Outport
  attitude : Outport  Port=2
  control inputs : Outport  Port=3
  velocity : Outport  Port=4
  velocity_0 : Outport  Port=5
  Vpsi : Outport  Port=6
  dot : Outport  Port=7
  wires:
  kinematic(NED)_psi/4 -> velocity_0/1
  Manual Switch/1 -> kinematic(NED)_psi/3, Mux5/3, Mux8/2  "psi"
  Mux8/1 -> Vpsi/1  "Vpsi"
  Airspeed Hold System/3 -> Mux7/1
  Mux7/1 -> dot/1  "dot"
  "Course error constraint [-pi, pi]1"/1(err_course) -> Product/1
  psi_c/1 -> Plus7/1, Plus5/1
  Plus7/1 -> "Course error constraint [-pi, pi]1"/1("err_course ")
  Integrator/1 -> Plus7/2, Manual Switch/2
  Product/1 -> Integrator/1, Mux7/2
  a_course/1 -> Product/2
  "Course error constraint [-pi, pi]"/1(err_course) -> Manual Switch2/1
  Mux4/1 -> velocity/1  "velocity"
  Manual Switch2/1 -> Kp_course/1, Ki_course/1, Derivative1/1
  wind/1 -> kinematic(NED)_psi/4
  Roll Hold System/1 -> Product1/2, Mux5/1  "phi"
  Kd_course/1 -> Plus3/3
  Mux5/1 -> attitude/1  "attitude"
  Plus2/1 -> Mux1/2  "Va_c"
  Mux6/1 -> control inputs/1  "control_inputs"
  kinematic(NED)_psi/5 -> Mux4/2
  Mux1/1 -> Va0 vs. Va/1
  Plus4/1 -> Product2/1, kinematic(NED)_psi/1, Mux4/1, Mux8/1, Mux1/1  "Va"
  Plus3/1 -> Roll Hold System/1
  Plus5/1 -> "Course error constraint [-pi, pi]"/1("err_course "), Manual Switch2/2  "err_course"
  Product2/1 -> Product1/1
  Kp_course/1 -> Plus3/2
  Product1/1 -> Integrator2/1
  Ki_course/1 -> Integrator3/1
  Integrator2/1 -> Plus5/2, Manual Switch/1  "psi"
  Mux3/1 -> position/1  "position"
  delta_t_star/1 -> Plus6/1
  Airspeed Hold System/1 -> Va_bar/1, Plus4/1  "Va_bar"
  Plus6/1 -> Mux6/1  "delta_t"
  "Pitch Hold System "/2 -> Mux6/2  "delta_e"
  Airspeed Hold System/2 -> Plus6/2  "delta_t_bar"
  Roll Hold System/2 -> Mux6/3  "delta_a"
  Va_bar_c/1 -> Airspeed Hold System/1, Plus2/2
  theta_c/1 -> "Pitch Hold System "/1
  kinematic(NED)_psi/2 -> Mux3/2  "y"
  "Pitch Hold System "/1 -> theta/1, kinematic(NED)_psi/2, Mux5/2  "theta"
  Va0/1 -> Plus4/2, Plus2/1
  Constant/1 -> Product2/2
  Derivative1/1 -> Kd_course/1
  kinematic(NED)_psi/1 -> Mux3/1  "x"
  kinematic(NED)_psi/3 -> Mux3/3  "z"
  Integrator3/1 -> Plus3/1
  kinematic(NED)_psi/6 -> Mux5/4
  kinematic(NED)_psi/7 -> Mux5/5

== system Fixed_Wing/Pitch Hold System  ==
  theta_c : Inport
  Constant : Constant  Value=1.57
  Derivative : Derivative
  Integrator : Integrator  InitialCondition=init.theta0
  Kd_theta : Gain  Gain=k_theta.Kd
  Kp_theta : Gain  Gain=k_theta.Kp
  Manual Switch : ManualSwitch  CurrentSetting=0
  Manual Switch1 : ManualSwitch  CurrentSetting=0
  Manual Switch2 : ManualSwitch
  Plus1 : Sum  Inputs=+-
  Plus2 : Sum  Inputs=+-
  Saturation : Saturate  UpperLimit=X8.delta.e_max  LowerLimit=X8.delta.e_min
  system1 : TransferFcn  Numerator=X8_lon_de_q_tf.Numerator{1,1}  Denominator=X8_lon_de_q_tf.Denominator{1,1}
  theta : Outport
  delta_e : Outport  Port=2
  wires:
  system1/1 -> Manual Switch1/2, Integrator/1  "q"
  Plus2/1 -> Manual Switch2/2, Saturation/1
  Kp_theta/1 -> Plus2/1
  Plus1/1 -> Kp_theta/1, Derivative/1  "err_theta"
  Integrator/1 -> theta/1, Plus1/2  "theta"
  Constant/1 -> Manual Switch/1
  Manual Switch/1 -> Plus1/1
  theta_c/1 -> Manual Switch/2
  Manual Switch1/1 -> Kd_theta/1
  Derivative/1 -> Manual Switch1/1
  Kd_theta/1 -> Plus2/2
  Manual Switch2/1 -> delta_e/1, system1/1  "delta_e"
  Saturation/1 -> Manual Switch2/1  "delta_e"

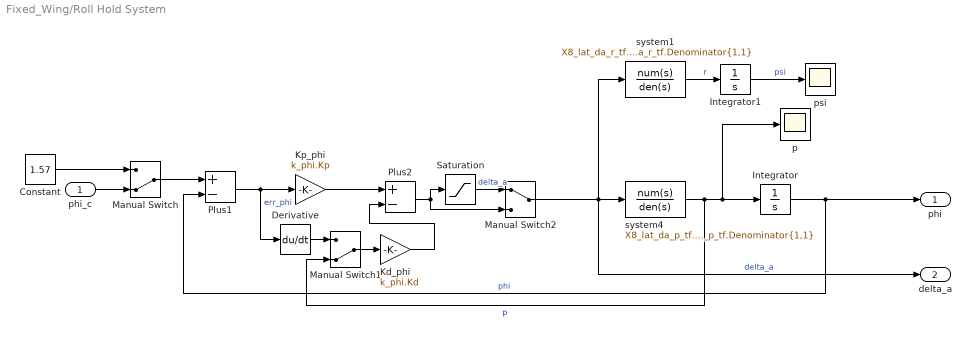
== system Fixed_Wing/Roll Hold System ==
  phi_c : Inport
  Constant : Constant  Value=1.57
  Derivative : Derivative
  Integrator : Integrator  InitialCondition=init.phi0
  Integrator1 : Integrator  InitialCondition=init.psi0
  Kd_phi : Gain  Gain=k_phi.Kd
  Kp_phi : Gain  Gain=k_phi.Kp
  Manual Switch : ManualSwitch  CurrentSetting=0
  Manual Switch1 : ManualSwitch  CurrentSetting=0
  Manual Switch2 : ManualSwitch
  Plus1 : Sum  Inputs=+-
  Plus2 : Sum  Inputs=+-
  Saturation : Saturate  UpperLimit=X8.delta.a_max  LowerLimit=X8.delta.a_min  LinearizeAsGain=off
  p : Scope
  psi : Scope
  system1 : TransferFcn  Numerator=X8_lat_da_r_tf.Numerator{1,1}  Denominator=X8_lat_da_r_tf.Denominator{1,1}
  system4 : TransferFcn  Numerator=X8_lat_da_p_tf.Numerator{1,1}  Denominator=X8_lat_da_p_tf.Denominator{1,1}
  phi : Outport
  delta_a : Outport  Port=2
  wires:
  system4/1 -> Manual Switch1/2, p/1, Integrator/1  "p"
  Plus2/1 -> Manual Switch2/2, Saturation/1
  Kp_phi/1 -> Plus2/1
  Plus1/1 -> Kp_phi/1, Derivative/1  "err_phi"
  Integrator/1 -> phi/1, Plus1/2  "phi"
  Constant/1 -> Manual Switch/1
  Manual Switch/1 -> Plus1/1
  phi_c/1 -> Manual Switch/2
  Manual Switch1/1 -> Kd_phi/1
  Derivative/1 -> Manual Switch1/1
  Kd_phi/1 -> Plus2/2
  Manual Switch2/1 -> delta_a/1, system4/1, system1/1  "delta_a"
  system1/1 -> Integrator1/1  "r"
  Integrator1/1 -> psi/1  "psi"
  Saturation/1 -> Manual Switch2/1  "delta_a"

== system Fixed_Wing/Wind model ==
  Manual Switch : ManualSwitch
  Manual Switch1 : ManualSwitch
  Manual Switch2 : ManualSwitch  CurrentSetting=0
  Non-steady wind gust : Subsystem
  Plus : Sum  Inputs=+++
  "Steady wind " : Subsystem
  Steady wind gust : Subsystem
  no wind : Subsystem
  wind : Outport
  wires:
  no wind/1(wind) -> Manual Switch2/2, Manual Switch/2, Manual Switch1/2
  Plus/1 -> wind/1  "wind"
  Steady wind gust/1(wgs) -> Manual Switch1/1  "wgs"
  Manual Switch1/1 -> Plus/2
  Manual Switch2/1 -> Plus/3
  Non-steady wind gust/1(wgn) -> Manual Switch2/1  "wgn"
  "Steady wind "/1(ws) -> Manual Switch/1  "ws"
  Manual Switch/1 -> Plus/1

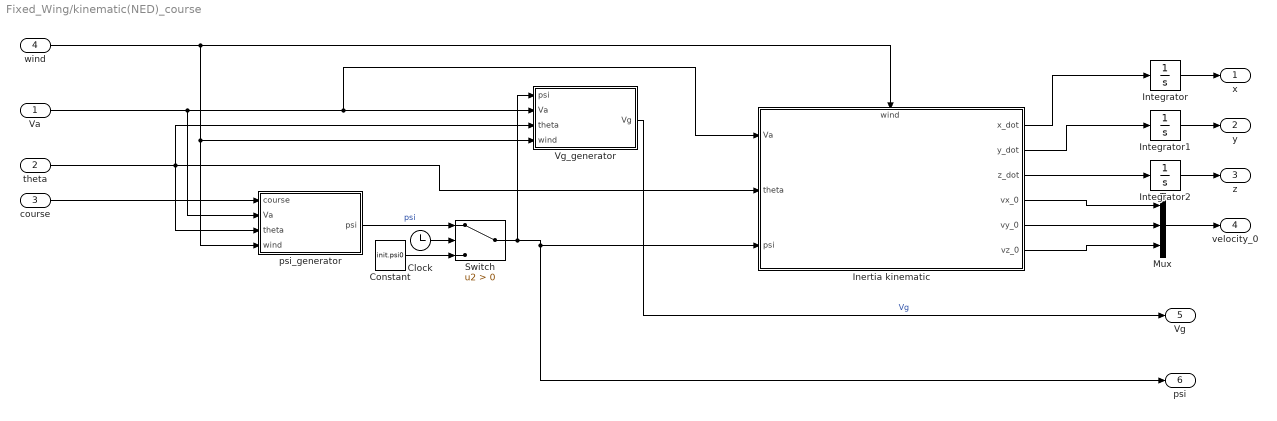
== system Fixed_Wing/kinematic(NED)_course ==
  Va : Inport
  theta : Inport  Port=2
  course : Inport  Port=3
  wind : Inport  Port=4
  Clock : Clock
  Constant : Constant  Value=init.psi0
  Inertia kinematic : Subsystem
      settings: PortSchema="{\"entries\":[{\"content\":{\"sides\":[{\"content\":{\"connectorIds\":[\"In1\",\"In2\",\"In3\"]},\"type\":\"ConnectorPlacement.EquallySpacedRectSide\",\"uuid\":\"18991cbd-8d8f-4668-8054-d56b6b4d2674\"},{\"content\":{\"connectorIds\":[\"Out1\",\"Out2\",\"Out3\",\"Out4\",\"Out5\",\"Out6\"],\"side\":\"RIGHT\"},\"type\":\"ConnectorPlacement.EquallySpacedRectSide\",\"uuid\":\"98d568d4-17ea-4287-b7bc-cb3e53942fc3\"},{\"content\":{\"connectorIds\":[\"In4\"],\"side\":\"TOP\"},\"type\":\"ConnectorPlacement.EquallySpacedRectSide\",\"uuid\":\"972ca0ea-c255-483c-a17b-ab0326bdc39e\"}]},\"type\":\"ConnectorPlacement.EquallySpacedConnector\",\"uuid\":\"0db01b3b-f146-4ef8-8588-0b44af2f41d6\"}],\"packageUris\":[\"http://schema.mathworks.com/mf0/Connector/R2020b\"],\"version\":\"1.0\"}"
  Integrator : Integrator  InitialCondition=init.x0
  Integrator1 : Integrator  InitialCondition=init.y0
  Integrator2 : Integrator  InitialCondition=init.z0
  Mux : Mux  Inputs=3
  Switch : Switch  Criteria=u2 > Threshold  SaturateOnIntegerOverflow=off  InputSameDT=off
  Vg_generator : MATLAB Function  TreatAsAtomicUnit=on
  "psi_generator " : MATLAB Function  TreatAsAtomicUnit=on
  x : Outport
  y : Outport  Port=2
  z : Outport  Port=3
  velocity_0 : Outport  Port=4
  Vg : Outport  Port=5
  psi : Outport  Port=6
  wires:
  Integrator2/1 -> z/1
  Integrator/1 -> x/1
  Integrator1/1 -> y/1
  Va/1 -> Vg_generator/2(Va), Inertia kinematic/1(Va), "psi_generator "/2(Va)
  course/1 -> "psi_generator "/1(course)
  theta/1 -> Inertia kinematic/2(theta), Vg_generator/3(theta), "psi_generator "/3(theta)
  wind/1 -> Inertia kinematic/4(wind), Vg_generator/4(wind), "psi_generator "/4(wind)
  Vg_generator/1(Vg) -> Vg/1  "Vg"
  Inertia kinematic/1(x_dot) -> Integrator/1
  Inertia kinematic/2(y_dot) -> Integrator1/1
  Inertia kinematic/3(z_dot) -> Integrator2/1
  Switch/1 -> Vg_generator/1(psi), Inertia kinematic/3(psi), psi/1
  Clock/1 -> Switch/2
  "psi_generator "/1(psi) -> Switch/1  "psi"
  Constant/1 -> Switch/3
  Inertia kinematic/4(vx_0) -> Mux/1
  Inertia kinematic/5(vy_0) -> Mux/2
  Inertia kinematic/6(vz_0) -> Mux/3
  Mux/1 -> velocity_0/1

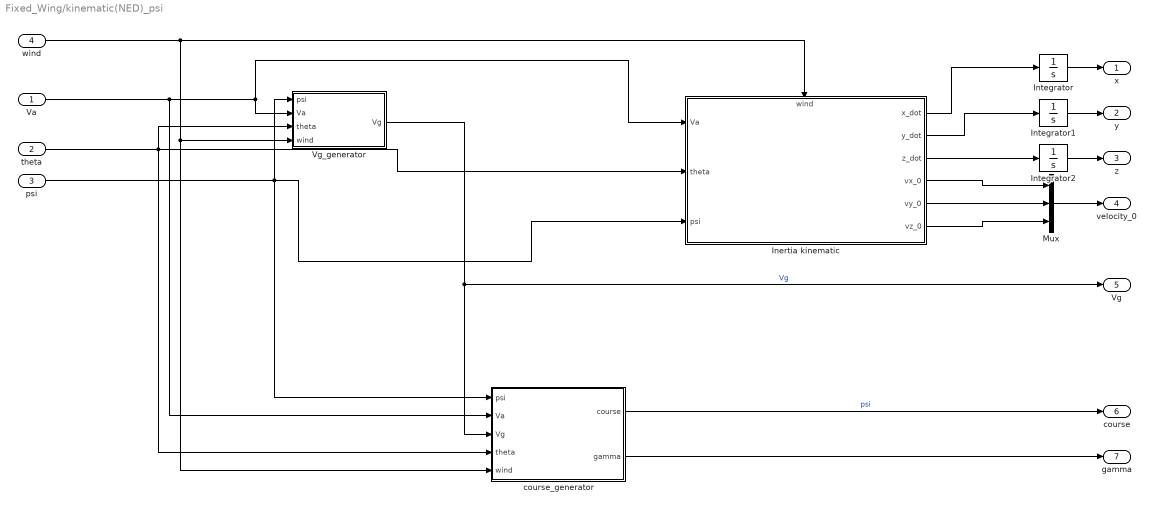
== system Fixed_Wing/kinematic(NED)_psi ==
  Va : Inport
  theta : Inport  Port=2
  psi : Inport  Port=3
  wind : Inport  Port=4
  Inertia kinematic : Subsystem
      settings: PortSchema="{\"entries\":[{\"content\":{\"sides\":[{\"content\":{\"connectorIds\":[\"In1\",\"In2\",\"In3\"]},\"type\":\"ConnectorPlacement.EquallySpacedRectSide\",\"uuid\":\"18991cbd-8d8f-4668-8054-d56b6b4d2674\"},{\"content\":{\"connectorIds\":[\"Out1\",\"Out2\",\"Out3\",\"Out4\",\"Out5\",\"Out6\"],\"side\":\"RIGHT\"},\"type\":\"ConnectorPlacement.EquallySpacedRectSide\",\"uuid\":\"98d568d4-17ea-4287-b7bc-cb3e53942fc3\"},{\"content\":{\"connectorIds\":[\"In4\"],\"side\":\"TOP\"},\"type\":\"ConnectorPlacement.EquallySpacedRectSide\",\"uuid\":\"972ca0ea-c255-483c-a17b-ab0326bdc39e\"}]},\"type\":\"ConnectorPlacement.EquallySpacedConnector\",\"uuid\":\"0db01b3b-f146-4ef8-8588-0b44af2f41d6\"}],\"packageUris\":[\"http://schema.mathworks.com/mf0/Connector/R2020b\"],\"version\":\"1.0\"}"
  Integrator : Integrator  InitialCondition=init.x0
  Integrator1 : Integrator  InitialCondition=init.y0
  Integrator2 : Integrator  InitialCondition=init.z0
  Mux : Mux  Inputs=3
  Vg_generator : MATLAB Function  TreatAsAtomicUnit=on
  "course_generator " : MATLAB Function  TreatAsAtomicUnit=on
  x : Outport
  y : Outport  Port=2
  z : Outport  Port=3
  velocity_0 : Outport  Port=4
  Vg : Outport  Port=5
  course : Outport  Port=6
  gamma : Outport  Port=7
  wires:
  Mux/1 -> velocity_0/1
  Inertia kinematic/6(vz_0) -> Mux/3
  Inertia kinematic/5(vy_0) -> Mux/2
  Inertia kinematic/4(vx_0) -> Mux/1
  psi/1 -> Inertia kinematic/3(psi), "course_generator "/1(psi), Vg_generator/1(psi)
  Inertia kinematic/3(z_dot) -> Integrator2/1
  Inertia kinematic/2(y_dot) -> Integrator1/1
  Inertia kinematic/1(x_dot) -> Integrator/1
  Vg_generator/1(Vg) -> Vg/1, "course_generator "/3(Vg)  "Vg"
  wind/1 -> "course_generator "/5(wind), Vg_generator/4(wind), Inertia kinematic/4(wind)
  theta/1 -> "course_generator "/4(theta), Vg_generator/3(theta), Inertia kinematic/2(theta)
  Va/1 -> "course_generator "/2(Va), Inertia kinematic/1(Va), Vg_generator/2(Va)
  Integrator1/1 -> y/1
  Integrator/1 -> x/1
  Integrator2/1 -> z/1
  "course_generator "/1(course) -> course/1  "psi"
  "course_generator "/2(gamma) -> gamma/1

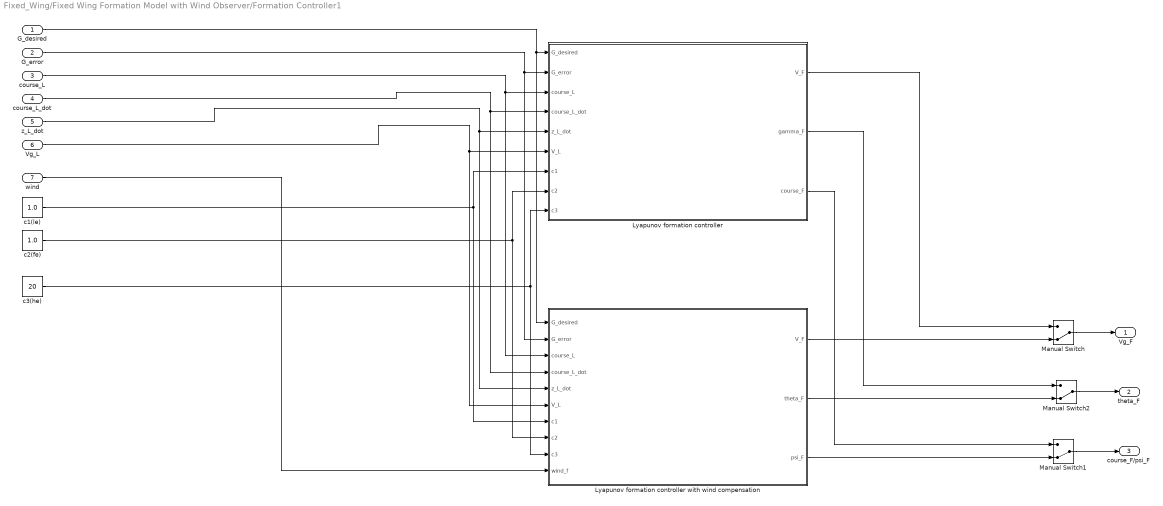
== system Fixed_Wing/Fixed Wing Formation Model with Wind Observer/Formation Controller1 ==
  G_desired : Inport
  G_error : Inport  Port=2
  course_L : Inport  Port=3
  course_L_dot : Inport  Port=4
  z_L_dot : Inport  Port=5
  Vg_L : Inport  Port=6
  wind : Inport  Port=7
  Lyapunov formation controller : MATLAB Function  TreatAsAtomicUnit=on
  Lyapunov formation controller with wind compensation : MATLAB Function  TreatAsAtomicUnit=on
  Manual Switch : ManualSwitch  CurrentSetting=0
  Manual Switch1 : ManualSwitch  CurrentSetting=0
  Manual Switch2 : ManualSwitch  CurrentSetting=0
  c1(le) : Constant  Value=1.0
  c2(fe) : Constant  Value=1.0
  c3(he) : Constant  Value=20
  Vg_F : Outport
  theta_F : Outport  Port=2
  course_F/psi_F : Outport  Port=3
  wires:
  c1(le)/1 -> Lyapunov formation controller with wind compensation/7(c1), Lyapunov formation controller/7(c1)
  c2(fe)/1 -> Lyapunov formation controller with wind compensation/8(c2), Lyapunov formation controller/8(c2)
  G_desired/1 -> Lyapunov formation controller with wind compensation/1(G_desired), Lyapunov formation controller/1(G_desired)
  course_L_dot/1 -> Lyapunov formation controller/4(course_L_dot), Lyapunov formation controller with wind compensation/4(course_L_dot)
  course_L/1 -> Lyapunov formation controller/3(course_L), Lyapunov formation controller with wind compensation/3(course_L)
  Vg_L/1 -> Lyapunov formation controller/6(V_L), Lyapunov formation controller with wind compensation/6(V_L)
  Lyapunov formation controller/1(V_F) -> Manual Switch/1
  Manual Switch/1 -> Vg_F/1
  Manual Switch1/1 -> course_F/psi_F/1
  Lyapunov formation controller/3(course_F) -> Manual Switch1/1
  wind/1 -> Lyapunov formation controller with wind compensation/10(wind_f)
  Lyapunov formation controller with wind compensation/1(V_F) -> Manual Switch/2
  Lyapunov formation controller with wind compensation/3(psi_F) -> Manual Switch1/2
  G_error/1 -> Lyapunov formation controller/2(G_error), Lyapunov formation controller with wind compensation/2(G_error)
  z_L_dot/1 -> Lyapunov formation controller/5(z_L_dot), Lyapunov formation controller with wind compensation/5(z_L_dot)
  c3(he)/1 -> Lyapunov formation controller/9(c3), Lyapunov formation controller with wind compensation/9(c3)
  Lyapunov formation controller/2(gamma_F) -> Manual Switch2/1
  Lyapunov formation controller with wind compensation/2(theta_F) -> Manual Switch2/2
  Manual Switch2/1 -> theta_F/1

== system Fixed_Wing/Fixed Wing Formation Model with Wind Observer/Formation Error1 ==
  G_desired : Inport
  course_L : Inport  Port=2
  position_L : Inport  Port=3
  position_F : Inport  Port=4
  "Geometry error " : MATLAB Function  TreatAsAtomicUnit=on
  G_error : Outport
  wires:
  G_desired/1 -> "Geometry error "/1(G_desired)
  course_L/1 -> "Geometry error "/2(course_L)
  position_L/1 -> "Geometry error "/3(position_L)
  position_F/1 -> "Geometry error "/4(position_F)
  "Geometry error "/1(G_error) -> G_error/1

== system Fixed_Wing/Fixed Wing Formation Model with Wind Observer/Wind Observer ==
  position : Inport
  velocity_0 : Inport  Port=2
  Constant : Constant
  Integrator : Integrator
  Integrator1 : Integrator
  Minus : Sum  Inputs=+-
  Position estimation : MATLAB Function  TreatAsAtomicUnit=on
  Wind acceleration estimation : MATLAB Function  TreatAsAtomicUnit=on
  position_hat : Outport
  w_hat : Outport  Port=2
  wires:
  Position estimation/1(velcocity_hat) -> Integrator1/1
  position/1 -> Minus/2
  Minus/1 -> Position estimation/3(sigma), Wind acceleration estimation/2(sigma)
  Wind acceleration estimation/1(w_a_hat) -> Integrator/1
  Constant/1 -> Position estimation/1(L), Wind acceleration estimation/1(L)
  Integrator1/1 -> Minus/1, position_hat/1
  Integrator/1 -> w_hat/1, Position estimation/2(w_hat)
  velocity_0/1 -> Position estimation/4(velocity_0)

== system Fixed_Wing/Wind model/Non-steady wind gust ==
  Band-Limited White Noise : simulink/Sources/Band-Limited White Noise  Cov=[0.1]  Ts=0.1  seed=[23341]
  Band-Limited White Noise1 : simulink/Sources/Band-Limited White Noise  Cov=[0.1]  Ts=0.1  seed=[23341]
  Mux : Mux  Inputs=3
  wd : Constant  Value=0
  wgn : Outport
  wires:
  wd/1 -> Mux/3  "wd"
  Mux/1 -> wgn/1  "ws"
  Band-Limited White Noise/1 -> Mux/1
  Band-Limited White Noise1/1 -> Mux/2

== system Fixed_Wing/Wind model/Steady wind  ==
  Clock : Clock
  Constant : Constant  Value=env.w.dir
  Constant1 : Constant
  Constant2 : Constant  Value=env.w.s
  Cos : Trigonometry  Operator=cos
  Divide : Product  Inputs=**
  Gain : Gain  Gain=-1
  Gain1 : Gain  Gain=-2
  Math Function : Math
  Mux : Mux  Inputs=3
  Plus : Sum  Inputs=+-
  Product : Product
  Product1 : Product
  Sin : Trigonometry
  wd : Constant  Value=0
  ws : Outport
  wires:
  wd/1 -> Mux/3  "wd"
  Mux/1 -> ws/1  "ws"
  Product1/1 -> Mux/1  "wn"
  Product/1 -> Mux/2  "we"
  Constant/1 -> Sin/1, Cos/1
  Sin/1 -> Product/1
  Cos/1 -> Product1/1
  Gain/1 -> Product1/2, Product/2
  Clock/1 -> Gain1/1
  Gain1/1 -> Math Function/1
  Math Function/1 -> Plus/2
  Constant1/1 -> Plus/1
  Constant2/1 -> Divide/1
  Plus/1 -> Divide/2
  Divide/1 -> Gain/1

== system Fixed_Wing/Wind model/Steady wind gust ==
  Clock : Clock
  Clock1 : Clock
  Constant : Constant
  Gain : Gain  Gain=0.2
  Gain1 : Gain  Gain=0.2
  Gain2 : Gain
  Gain3 : Gain
  Gain4 : Gain  Gain=0.5
  Mux : Mux  Inputs=3
  Plus : Sum  Inputs=+-
  Sin : Trigonometry
  Sin1 : Trigonometry  Operator=cos
  wgs : Outport
  wires:
  Mux/1 -> wgs/1  "ws"
  Sin/1 -> Gain4/1, Gain2/1  "wn"
  Sin1/1 -> Plus/1
  Clock/1 -> Gain1/1
  Clock1/1 -> Gain/1
  Gain/1 -> Sin1/1
  Gain1/1 -> Sin/1
  Gain2/1 -> Mux/1
  Gain3/1 -> Mux/2  "we"
  Plus/1 -> Gain3/1
  Constant/1 -> Plus/2
  Gain4/1 -> Mux/3  "wd"

== system Fixed_Wing/Wind model/no wind ==
  Mux : Mux  Inputs=3
  wd : Constant  Value=0
  we : Constant  Value=0
  wn : Constant  Value=0
  wind : Outport
  wires:
  wd/1 -> Mux/3  "wd"
  Mux/1 -> wind/1
  wn/1 -> Mux/1  "wn"
  we/1 -> Mux/2  "we"

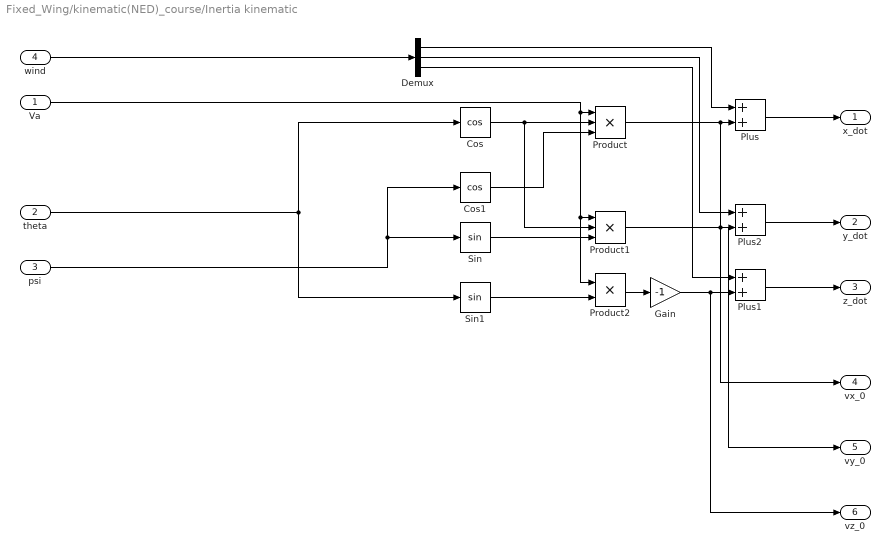
== system Fixed_Wing/kinematic(NED)_course/Inertia kinematic ==
  Va : Inport
  theta : Inport  Port=2
  psi : Inport  Port=3
  wind : Inport  Port=4
  Cos : Trigonometry  Operator=cos
  Cos1 : Trigonometry  Operator=cos
  Demux : Demux  Outputs=3
  Gain : Gain  Gain=-1
  Plus : Sum
  Plus1 : Sum
  Plus2 : Sum
  Product : Product  Inputs=3
  Product1 : Product  Inputs=3
  Product2 : Product
  Sin : Trigonometry
  Sin1 : Trigonometry
  x_dot : Outport
  y_dot : Outport  Port=2
  z_dot : Outport  Port=3
  vx_0 : Outport  Port=4
  vy_0 : Outport  Port=5
  vz_0 : Outport  Port=6
  wires:
  Va/1 -> Product2/1, Product1/1, Product/1
  Demux/3 -> Plus1/1
  Demux/2 -> Plus2/1
  Demux/1 -> Plus/1
  Plus/1 -> x_dot/1
  Plus2/1 -> y_dot/1
  Plus1/1 -> z_dot/1
  Sin1/1 -> Product2/2
  Cos/1 -> Product/2, Product1/2
  Product2/1 -> Gain/1
  Sin/1 -> Product1/3
  Cos1/1 -> Product/3
  theta/1 -> Cos/1, Sin1/1
  psi/1 -> Cos1/1, Sin/1
  wind/1 -> Demux/1
  Gain/1 -> Plus1/2, vz_0/1
  Product1/1 -> vy_0/1, Plus2/2
  Product/1 -> vx_0/1, Plus/2

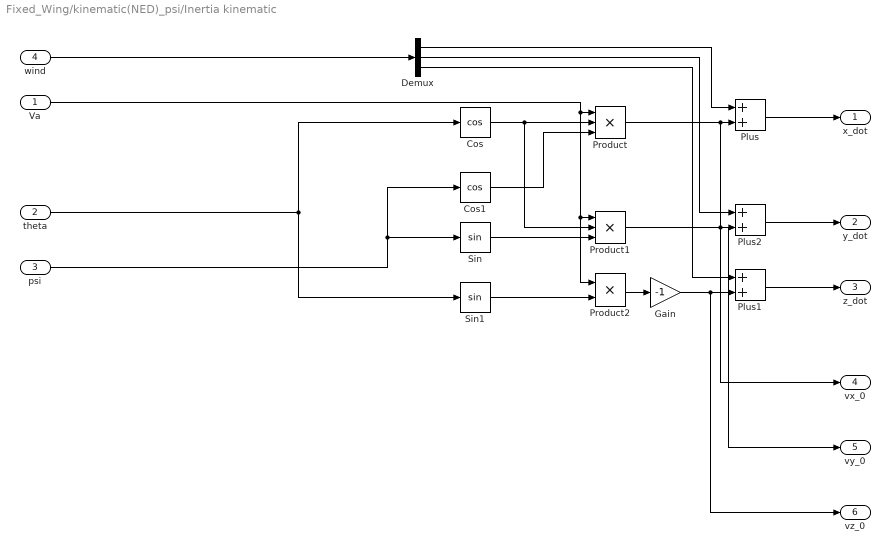
== system Fixed_Wing/kinematic(NED)_psi/Inertia kinematic ==
  Va : Inport
  theta : Inport  Port=2
  psi : Inport  Port=3
  wind : Inport  Port=4
  Cos : Trigonometry  Operator=cos
  Cos1 : Trigonometry  Operator=cos
  Demux : Demux  Outputs=3
  Gain : Gain  Gain=-1
  Plus : Sum
  Plus1 : Sum
  Plus2 : Sum
  Product : Product  Inputs=3
  Product1 : Product  Inputs=3
  Product2 : Product
  Sin : Trigonometry
  Sin1 : Trigonometry
  x_dot : Outport
  y_dot : Outport  Port=2
  z_dot : Outport  Port=3
  vx_0 : Outport  Port=4
  vy_0 : Outport  Port=5
  vz_0 : Outport  Port=6
  wires:
  Product/1 -> Plus/2, vx_0/1
  Product1/1 -> Plus2/2, vy_0/1
  Gain/1 -> vz_0/1, Plus1/2
  wind/1 -> Demux/1
  psi/1 -> Sin/1, Cos1/1
  theta/1 -> Sin1/1, Cos/1
  Cos1/1 -> Product/3
  Sin/1 -> Product1/3
  Product2/1 -> Gain/1
  Cos/1 -> Product1/2, Product/2
  Sin1/1 -> Product2/2
  Plus1/1 -> z_dot/1
  Plus2/1 -> y_dot/1
  Plus/1 -> x_dot/1
  Demux/1 -> Plus/1
  Demux/2 -> Plus2/1
  Demux/3 -> Plus1/1
  Va/1 -> Product/1, Product1/1, Product2/1

== matlab function Fixed_Wing/Fixed Wing Model(Va,course,theta)/Course error constraint [-pi, pi] ==
  data: err_course input; err_course output
function err_course = constraint(err_course)
    while err_course < -pi
        err_course = err_course + 2*pi;
        % err_lt_mpi = err_course
        % display("err < -pi", err_course);
    end
    while err_course > pi
        err_course = err_course - 2*pi;
        % err_gt_pi = err_course
        % display("err > pi", err_course);
    end
end

== matlab function Fixed_Wing/Fixed Wing Model(Va,course,theta)/Course error constraint [-pi, pi]1 ==
  data: err_course input; err_course output
function err_course = constraint(err_course)
    while err_course < -pi
        err_course = err_course + 2*pi;
        % err_lt_mpi = err_course
        % display("err < -pi", err_course);
    end
    while err_course > pi
        err_course = err_course - 2*pi;
        % err_gt_pi = err_course
        % display("err > pi", err_course);
    end
end

== matlab function Fixed_Wing/Fixed Wing Formation Model with Wind Observer/Formation Controller1/Lyapunov formation controller ==
  data: G_desired input; G_error input; course_L input; course_L_dot input; z_L_dot input; V_L input; c1 input; c2 input; V_F output; gamma_F output size=1; c3 input; course_F output
function [V_F, gamma_F, course_F] = lyapunov_formation(G_desired, G_error, course_L, course_L_dot, z_L_dot, V_L,c1, c2, c3)
    lc = G_desired(1);
    fc = G_desired(2);
    hc = G_desired(3);
    le = G_error(1);
    fe = G_error(2);
    he = G_error(3);

    

    
    % course_F = atan2(-c1*le-course_L_dot*(fe+fc), c2*fe-course_L_dot*(le+lc)+V_L)+course_L;
    % V_F = sqrt((c1*le+course_L_dot*(fe+fc))^2+(c2*fe-course_L_dot*(le+lc)+V_L)^2);

    course_F = atan2(-c1*le-course_L_dot*fc, c2*fe-course_L_dot*lc+V_L)+course_L;
    V_F = sqrt((c1*le+course_L_dot*fc)^2+(c2*fe-course_L_dot*lc+V_L)^2);
    
    % ensure that the value in asin funtion fall between [-1,1]
    gam = c3*he+z_L_dot;
    if gam > V_F
        gam = V_F;
    elseif gam < -V_F
        gam = -V_F;
    end

    gamma_F = asin(gam/V_F);

end

== matlab function Fixed_Wing/Fixed Wing Formation Model with Wind Observer/Formation Controller1/Lyapunov formation controller with wind compensation ==
  data: G_desired input; G_error input; course_L input; course_L_dot input; z_L_dot input; V_L input; V_F output; theta_F output size=1; c1 input; c2 input; c3 input; psi_F output; wind_f input
function [V_F, theta_F, psi_F] = lyapunov_formation(G_desired, G_error, course_L, course_L_dot, z_L_dot, V_L,c1, c2, c3, wind_f)
    lc = G_desired(1);
    fc = G_desired(2);
    hc = G_desired(3);
    le = G_error(1);
    fe = G_error(2);
    he = G_error(3);
    wl = wind_f(1);
    wf = wind_f(2);
    wh = wind_f(3);

    psi_F = atan2(-c1*le-course_L_dot*fc-wl, c2*fe-course_L_dot*lc+V_L+wf)+course_L;
    V_F = sqrt((c1*le+course_L_dot*fc+wl)^2+(c2*fe-course_L_dot*lc+V_L+wf)^2);

    % ensure that the value in asin funtion fall between [-1,1]
    gam = c3*he-z_L_dot+wh;
    if gam > V_F
        gam = V_F;
    elseif gam < -V_F
        gam = -V_F;
    end

    theta_F = asin(gam/V_F);
end
